simulink library "sm_ball_bearing_testrig_lib"  (R2019a)
settings: Solver=VariableStepAuto  StartTime=0.0  StopTime=10.0  RelTol=1e-3
undefined symbols (not defined in the file): bearing, bearing_ball_cage_b, bearing_ball_clr, bearing_ball_mark_clr, bearing_ball_mark_opc, bearing_ball_opc, bearing_ball_preload, bearing_ball_rad, bearing_ball_rho, bearing_cage_clr, bearing_cage_loop_xc, bearing_cage_opc, bearing_cage_rad_ctr, bearing_cage_rho, bearing_cage_web_thk, bearing_cage_web_xc, bearing_ir_all, bearing_ir_xc, bearing_or_all, bearing_or_xc, X, Y, Z
libraries: $bdroot x26, sm_lib x25, Contact_Forces_Lib x2, nesl_utility x1
Description:
  | Copyright 2018-2019 The MathWorks, Inc.
settings Model: Creator=smiller  LastModifiedBy=smiller
settings DataIOCC: ReturnWorkspaceOutputs=off
settings DebuggingCC: PregeneratedLibrarySubsystemCodeDiagnostic=none  ArithmeticOperatorsInVariantConditions=warning
settings SFSimCC: SimUseLocalCustomCode=off
settings RTWCC: RTWUseLocalCustomCode=off

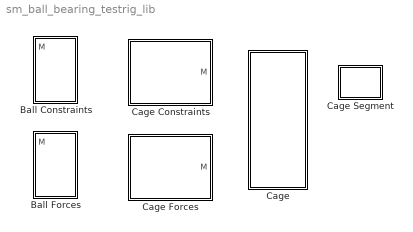
== system sm_ball_bearing_testrig_lib ==
  Ball Constraints : Subsystem  mask{ball_rad=0.005, ball_rho=7000, ball_cage_b=0, ball_clr=[0.6 0.6 0.6], ball_opc=1, mark_clr=[0.8 0.8 0.8], mark_opc=1, bearing_or=0.1, bearing_ir=0.05}
      mask prompts: ball_rad "Radius (m)"; ball_rho "Density (kg/m^3)"; ball_cage_b "Ball-Cage Viscous Friction (N*m/(deg/s))"; ball_clr "Color [R G B]"; ball_opc "Opacity (0-1)"; mark_clr "Color [R G B]"; mark_opc "Opacity (0-1)"; bearing_or "Bearing Outer Radius (m)"; bearing_ir "Bearing Inner Radius (m)"
      mask DialogControl cont_ball Prompt: Ball
      mask DialogControl cont_marking Prompt: Marking
      mask DialogControl cont_race Prompt: Race
      mask Display: image('sm_ball_bearing_testrig_ball_constraints_IMAGE.png');
  Ball Forces : Subsystem  mask{ball_rad=0.005, ball_rho=7000, ball_cage_b=0, ball_clr=[0.6 0.6 0.6], ball_opc=1, mark_clr=[0.8 0.8 0.8], mark_opc=1, bearing_or=0.1, bearing_ir=0.05, ball_k=1e5, ball_preload=5, ball_innerrace_overlap=0, ball_b=1e4, ball_muk=0.7, ball_mus=0.9, ball_vth=1e-3}
      mask prompts: ball_rad "Radius (m)"; ball_rho "Density (kg/m^3)"; ball_cage_b "Ball-Cage Viscous Friction (N*m/(deg/s))"; ball_clr "Color [RGB]"; ball_opc "Opacity (0-1)"; mark_clr "Color [RGB]"; mark_opc "Opacity (0-1)"; bearing_or "Bearing Outer Radius (m)"; bearing_ir "Bearing Inner Radius (m)"; ball_k "Stiffness (N/m)"; ball_preload "Preload Force Per Ball (N)"; ball_innerrace_overlap "Clearance (m)"; ball_b "Damping (N/(m/s))"; ball_muk "Coefficient of Kinetic Friction"; ball_mus "Coefficient of Static Friction"; ball_vth "Velocity Threshold (m/s)"
      mask init:
      | % Convert preload force to interference 
      | % for use in inner race contact force
      | % Positive interference = initial penetration
      | ball_innerrace_overlap = ball_preload/ball_k*2;
      mask DialogControl cont_ball Prompt: Ball
      mask DialogControl cont_marking Prompt: Marking
      mask DialogControl cont_race Prompt: Race
      mask DialogControl cont_forces Prompt: Forces
      mask Display: image('sm_ball_bearing_testrig_ball_forces_IMAGE.png');
  Cage : Subsystem
      mask Display: image('sm_ball_bearing_testrig_cage_IMAGE.png')
  Cage Constraints : Subsystem  Tag=PublishSubsystem  mask{ball_rad_all=bearing_ball_rad, ball_rho_all=bearing_ball_rho, ball_cage_b_all=bearing_ball_cage_b, ball_clr_all=bearing_ball_clr, ball_opc_all=bearing_ball_opc, ball_mark_clr_all=bearing_ball_mark_clr, ball_mark_opc_all=bearing_ball_mark_opc, bearing_or_all=max(bearing_or_xc(:,1))*2, bearing_ir_all=min(bearing_ir_xc(:,1))*2}
      mask prompts: ball_rad_all "Radius (m)"; ball_rho_all "Density (kg/m^3)"; ball_cage_b_all "Ball-Cage Viscous Friction (N*m/(deg/s))"; ball_clr_all "Color [R G B]"; ball_opc_all "Opacity (0-1)"; ball_mark_clr_all "Color [R G B]"; ball_mark_opc_all "Opacity (0-1)"; bearing_or_all "Bearing Outer Radius (m)"; bearing_ir_all "Bearing Inner Radius (m)"
      mask DialogControl cont_ball Prompt: Ball
      mask DialogControl cont_marking Prompt: Marking
      mask DialogControl cont_race_all Prompt: Race
      mask Display: image('sm_ball_bearing_testrig_cage_constraints_IMAGE.png');
  Cage Forces : Subsystem  Tag=PublishSubsystem  mask{ball_rad_all=bearing_ball_rad, ball_rho_all=bearing_ball_rho, ball_cage_b_all=bearing_ball_cage_b, ball_clr_all=bearing_ball_clr, ball_opc_all=bearing_ball_opc, ball_mark_clr_all=bearing_ball_mark_clr, ball_mark_opc_all=bearing_ball_mark_opc, bearing_or_all=max(bearing_or_xc(:,1))*2, bearing_ir_all=min(bearing_ir_xc(:,1))*2, ball_k_all=1e5, ball_preload_all=bearing_ball_preload, ball_b_all=1e4, ball_muk_all=0.7, ball_mus_all=0.9, ball_vth_all=1e-3}
      mask prompts: ball_rad_all "Radius (m)"; ball_rho_all "Density (kg/m^3)"; ball_cage_b_all "Ball-Cage Viscous Friction (N*m/(deg/s))"; ball_clr_all "Color [R G B]"; ball_opc_all "Opacity (0-1)"; ball_mark_clr_all "Color [R G B]"; ball_mark_opc_all "Opacity (0-1)"; bearing_or_all "Bearing Outer Radius (m)"; bearing_ir_all "Bearing Inner Radius (m)"; ball_k_all "Stiffness (N/m)"; ball_preload_all "Preload Force Per Ball (N)"; ball_b_all "Damping (N/(m/s))"; ball_muk_all "Coefficient of Kinetic Friction"; ball_mus_all "Coefficient of Static Friction"; ball_vth_all "Velocity Threshold (m/s)"
      mask DialogControl cont_ball Prompt: Ball
      mask DialogControl cont_marking Prompt: Marking
      mask DialogControl cont_race_all Prompt: Race
      mask DialogControl cont_forces Prompt: Forces
      mask Display: image('sm_ball_bearing_testrig_cage_forces_IMAGE.png');
  Cage Segment : Subsystem  mask{cage_loop_xc=bearing_cage_loop_xc, cage_web_xc=bearing_cage_web_xc, cage_web_thk=bearing_cage_web_thk, cage_rad_ctr=bearing_cage_rad_ctr, cage_rho=bearing_cage_rho, cage_clr=bearing_cage_clr, cage_opc=bearing_cage_opc}
      mask prompts: cage_loop_xc "Cross Section for Loop [x y] (m)"; cage_web_xc "Cross Section for Web [x y] (m)"; cage_web_thk "Thickness of Web (m)"; cage_rad_ctr "Radius of Web Centerline (m)"; cage_rho "Density (kg/m^3)"; cage_clr "Color [RGB]"; cage_opc "Opacity"
      mask DialogControl cont_cage Prompt: Cage
      mask Display: image('sm_ball_bearing_testrig_cage_segment_IMAGE.png')

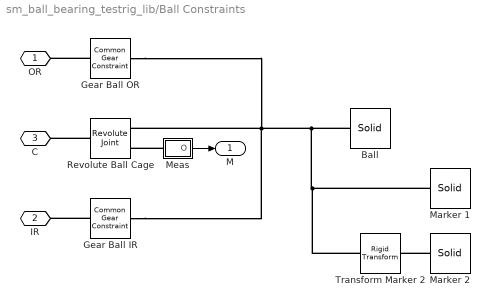
== system sm_ball_bearing_testrig_lib/Ball Constraints ==
  Ball : sm_lib/Body Elements/Solid  InertiaType=CalculateFromGeometry  Mass=1  MassUnits=kg  CenterOfMass=[0 0 0]  CenterOfMassUnits=m  MomentsOfInertia=[1 1 1]  MomentsOfInertiaUnits=kg*m^2  ProductsOfInertia=[1 1 1]  ProductsOfInertiaUnits=kg*m^2  BasedOnType=Density  Density=ball_rho  DensityUnits=kg/m^3  DoExposeReferenceFrame=on  SerializedFrames=<Frames/>  GraphicType=FromGeometry  MarkerShape=Sphere  MarkerSize=10  GraphicVisPropType=SimpleVisualProperties  GraphicDiffuseColor=ball_clr  GraphicSpecularColor=[0.5 0.5 0.5 1.0]  GraphicAmbientColor=[0.15 0.15 0.15 1.0]  GraphicEmissiveColor=[0.0 0.0 0.0 1.0]  GraphicShininess=75  GraphicOpacity=ball_opc  GeometryShape=Sphere  RectangleSize=[1 1]  RectangleSizeUnits=m  BrickDimensions=[1 1 1]  BrickDimensionUnits=m  CylinderRadius=1  CylinderRadiusUnits=m  CylinderLength=1  CylinderLengthUnits=m  SphereRadius=ball_rad  SphereRadiusUnits=m  EllipsoidRadii=[1 1 1]  EllipsoidRadiiUnits=m  ExtrusionCrossSection=[1 1; -1 1; -1 -1; 1 -1]  ExtrusionCrossSectionUnits=m  ExtrusionLength=1  ExtrusionLengthUnits=m  PolygonNumSides=3  PolygonOuterRadius=1  PolygonOuterRadiusUnits=m  ExtGeomFileType=STEP  ExtGeomFileUnits=m  RevolutionCrossSection=[1 1; 1 -1; 2 -1; 2 1]  RevolutionCrossSectionUnits=m  RevolutionExtent=Full  RevolutionAngle=180  RevolutionAngleUnits=deg
  Gear Ball IR : sm_lib/Gears and Couplings/Gears/Common Gear Constraint  GearType=External  SpecificationType=PitchCircleRadii  CenterDistance=20.0  CenterDistanceUnits=cm  GearRatio=1.0  BaseGearRadius=(bearing_or+bearing_ir)/4-ball_rad  BaseGearRadiusUnits=m  FollGearRadius=ball_rad  FollGearRadiusUnits=m  AssemblyGearRotation=Free
      settings: SourceProductName=Simscape Multibody  SourceProductBaseCode=MS
  Gear Ball OR : sm_lib/Gears and Couplings/Gears/Common Gear Constraint  GearType=Internal  SpecificationType=PitchCircleRadii  CenterDistance=20.0  CenterDistanceUnits=cm  GearRatio=1.0  BaseGearRadius=(bearing_or+bearing_ir)/4+ball_rad  BaseGearRadiusUnits=m  FollGearRadius=ball_rad  FollGearRadiusUnits=m  AssemblyGearRotation=Free
      settings: SourceProductName=Simscape Multibody  SourceProductBaseCode=MS
  Marker 1 : sm_lib/Body Elements/Solid  InertiaType=CalculateFromGeometry  Mass=1  MassUnits=kg  CenterOfMass=[0 0 0]  CenterOfMassUnits=m  MomentsOfInertia=[1 1 1]  MomentsOfInertiaUnits=kg*m^2  ProductsOfInertia=[1 1 1]  ProductsOfInertiaUnits=kg*m^2  BasedOnType=Density  Density=0  DensityUnits=kg/m^3  DoExposeReferenceFrame=on  SerializedFrames=<Frames/>  GraphicType=FromGeometry  MarkerShape=Sphere  MarkerSize=10  GraphicVisPropType=SimpleVisualProperties  GraphicDiffuseColor=mark_clr  GraphicSpecularColor=[0.5 0.5 0.5 1.0]  GraphicAmbientColor=[0.15 0.15 0.15 1.0]  GraphicEmissiveColor=[0.0 0.0 0.0 1.0]  GraphicShininess=75  GraphicOpacity=mark_opc  GeometryShape=GeneralSolidOfRevolution  RectangleSize=[1 1]  RectangleSizeUnits=m  BrickDimensions=[1 1 1]  BrickDimensionUnits=m  CylinderRadius=1  CylinderRadiusUnits=m  CylinderLength=1  CylinderLengthUnits=m  SphereRadius=1  SphereRadiusUnits=m  EllipsoidRadii=[1 1 1]  EllipsoidRadiiUnits=m  ExtrusionCrossSection=[1 1; -1 1; -1 -1; 1 -1]  ExtrusionCrossSectionUnits=m  ExtrusionLength=1  ExtrusionLengthUnits=m  PolygonNumSides=3  PolygonOuterRadius=1  PolygonOuterRadiusUnits=m  ExtGeomFileType=STEP  ExtGeomFileUnits=m  RevolutionCrossSection=[0.5 1; 0.5 -1; 0.7 -1; 0.7 1].*[ball_rad ball_rad*0.8]  RevolutionCrossSectionUnits=m  RevolutionExtent=Custom  RevolutionAngle=60  RevolutionAngleUnits=deg
  Marker 2 : sm_lib/Body Elements/Solid  InertiaType=CalculateFromGeometry  Mass=1  MassUnits=kg  CenterOfMass=[0 0 0]  CenterOfMassUnits=m  MomentsOfInertia=[1 1 1]  MomentsOfInertiaUnits=kg*m^2  ProductsOfInertia=[1 1 1]  ProductsOfInertiaUnits=kg*m^2  BasedOnType=Density  Density=0  DensityUnits=kg/m^3  DoExposeReferenceFrame=on  SerializedFrames=<Frames/>  GraphicType=FromGeometry  MarkerShape=Sphere  MarkerSize=10  GraphicVisPropType=SimpleVisualProperties  GraphicDiffuseColor=mark_clr  GraphicSpecularColor=[0.5 0.5 0.5 1.0]  GraphicAmbientColor=[0.15 0.15 0.15 1.0]  GraphicEmissiveColor=[0.0 0.0 0.0 1.0]  GraphicShininess=75  GraphicOpacity=mark_opc  GeometryShape=GeneralSolidOfRevolution  RectangleSize=[1 1]  RectangleSizeUnits=m  BrickDimensions=[1 1 1]  BrickDimensionUnits=m  CylinderRadius=1  CylinderRadiusUnits=m  CylinderLength=1  CylinderLengthUnits=m  SphereRadius=1  SphereRadiusUnits=m  EllipsoidRadii=[1 1 1]  EllipsoidRadiiUnits=m  ExtrusionCrossSection=[1 1; -1 1; -1 -1; 1 -1]  ExtrusionCrossSectionUnits=m  ExtrusionLength=1  ExtrusionLengthUnits=m  PolygonNumSides=3  PolygonOuterRadius=1  PolygonOuterRadiusUnits=m  ExtGeomFileType=STEP  ExtGeomFileUnits=m  RevolutionCrossSection=[0.5 1; 0.5 -1; 0.7 -1; 0.7 1].*[ball_rad ball_rad*0.8]  RevolutionCrossSectionUnits=m  RevolutionExtent=Custom  RevolutionAngle=60  RevolutionAngleUnits=deg
  Meas : Subsystem
  Revolute Ball Cage : sm_lib/Joints/Revolute Joint  SenseConstraintForce=off  SenseConstraintForceX=off  SenseConstraintForceY=off  SenseConstraintForceZ=off  SenseConstraintTorque=off  SenseConstraintTorqueX=off  SenseConstraintTorqueY=off  SenseConstraintTorqueZ=off  SenseTotalForce=off  SenseTotalForceX=off  SenseTotalForceY=off  SenseTotalForceZ=off  SenseTotalTorque=off  SenseTotalTorqueX=off  SenseTotalTorqueY=off  SenseTotalTorqueZ=off  CompositeWrenchDir=FollowerOnBase  CompositeWrenchFrame=BaseFrame  EquilibriumPosition=0  EquilibriumPositionUnits=deg  SpringStiffness=0  SpringStiffnessUnits=N*m/deg  DampingCoefficient=ball_cage_b  DampingCoefficientUnits=N*m/(deg/s)  TorqueActuationMode=NoTorque  MotionActuationMode=ComputedMotion  SensePosition=off  SenseVelocity=on  SenseAcceleration=off  SenseTorqueForce=off  SenseLowerLimitTorqueForce=off  SenseUpperLimitTorqueForce=off  LowerLimitSpecify=off  LowerLimitBound=-90  LowerLimitBoundUnits=deg  LowerLimitStiffness=1e4  LowerLimitStiffnessUnits=N*m/deg  LowerLimitDamping=10  LowerLimitDampingUnits=N*m/(deg/s)  LowerLimitTransitionRegionWidth=0.1  LowerLimitTransitionRegionWidthUnits=deg  UpperLimitSpecify=off  UpperLimitBound=90  UpperLimitBoundUnits=deg  UpperLimitStiffness=1e4  UpperLimitStiffnessUnits=N*m/deg  UpperLimitDamping=10  UpperLimitDampingUnits=N*m/(deg/s)  UpperLimitTransitionRegionWidth=0.1  UpperLimitTransitionRegionWidthUnits=deg  PositionTargetSpecify=off  PositionTargetPriority=High  PositionTargetValue=0  PositionTargetValueUnits=deg  VelocityTargetSpecify=off  VelocityTargetPriority=High  VelocityTargetValue=0  VelocityTargetValueUnits=deg/s
  Transform Marker 2 : sm_lib/Frames and Transforms/Rigid Transform  TranslationMethod=None  TranslationStandardOffset=0  TranslationLengthUnit=m  TranslationStandardAxis=+Z  TranslationCartesianOffset=[0 0 0]  TranslationROffset=0  TranslationROffsetUnits=m  TranslationZOffset=0  TranslationZOffsetUnits=m  TranslationThetaOffset=0  TranslationThetaOffsetUnits=deg  RotationMethod=StandardAxis  RotationAngleUnits=deg  RotationStandardAxis=+Z  RotationAngle=180  RotationArbitraryAxis=[0 0 1]  FollAlignAxisA=+X  BaseAlignAxisA=+Y  FollAlignAxisB=+Y  BaseAlignAxisB=+Z  RotationSequenceAxes=FollowerAxes  RotationSequence=XYX  RotationSequenceAngles=[0 0 0]  RotationSequenceAnglesUnits=deg  RotationMatrix=[1 0 0; 0 1 0; 0 0 1]
  OR : PMIOPort  Side=Right
  IR : PMIOPort  Port=2  Side=Right
  C : PMIOPort  Port=3  Side=Right
  M : Outport
  wires:
  Meas/1(O) -> M/1
  connections:
  Gear Ball OR/LConn1 -- OR/RConn1
  Gear Ball IR/LConn1 -- IR/RConn1
  Marker 1/RConn1 -- Ball/RConn1 -- Revolute Ball Cage/RConn1 -- Gear Ball OR/RConn1 -- Gear Ball IR/RConn1 -- Transform Marker 2/LConn1
  Revolute Ball Cage/LConn1 -- C/RConn1
  Marker 2/RConn1 -- Transform Marker 2/RConn1
  Meas/LConn1 -- Revolute Ball Cage/RConn2

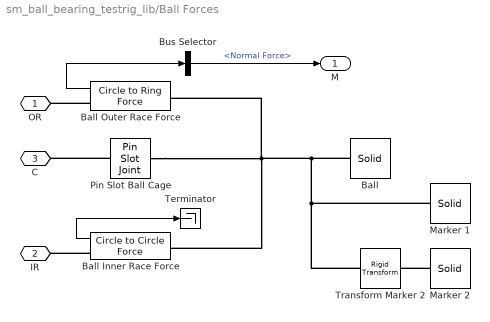
== system sm_ball_bearing_testrig_lib/Ball Forces ==
  Ball : sm_lib/Body Elements/Solid  InertiaType=CalculateFromGeometry  Mass=1  MassUnits=kg  CenterOfMass=[0 0 0]  CenterOfMassUnits=m  MomentsOfInertia=[1 1 1]  MomentsOfInertiaUnits=kg*m^2  ProductsOfInertia=[1 1 1]  ProductsOfInertiaUnits=kg*m^2  BasedOnType=Density  Density=ball_rho  DensityUnits=kg/m^3  DoExposeReferenceFrame=on  SerializedFrames=<Frames/>  GraphicType=FromGeometry  MarkerShape=Sphere  MarkerSize=10  GraphicVisPropType=SimpleVisualProperties  GraphicDiffuseColor=ball_clr  GraphicSpecularColor=[0.5 0.5 0.5 1.0]  GraphicAmbientColor=[0.15 0.15 0.15 1.0]  GraphicEmissiveColor=[0.0 0.0 0.0 1.0]  GraphicShininess=75  GraphicOpacity=ball_opc  GeometryShape=Sphere  RectangleSize=[1 1]  RectangleSizeUnits=m  BrickDimensions=[1 1 1]  BrickDimensionUnits=m  CylinderRadius=1  CylinderRadiusUnits=m  CylinderLength=1  CylinderLengthUnits=m  SphereRadius=ball_rad  SphereRadiusUnits=m  EllipsoidRadii=[1 1 1]  EllipsoidRadiiUnits=m  ExtrusionCrossSection=[1 1; -1 1; -1 -1; 1 -1]  ExtrusionCrossSectionUnits=m  ExtrusionLength=1  ExtrusionLengthUnits=m  PolygonNumSides=3  PolygonOuterRadius=1  PolygonOuterRadiusUnits=m  ExtGeomFileType=STEP  ExtGeomFileUnits=m  RevolutionCrossSection=[1 1; 1 -1; 2 -1; 2 1]  RevolutionCrossSectionUnits=m  RevolutionExtent=Full  RevolutionAngle=180  RevolutionAngleUnits=deg
  Ball Inner Race Force : Contact_Forces_Lib/2D/Circle to Circle Force  cirB_rad=(bearing_or+bearing_ir)/4-ball_rad+ball_innerrace_overlap  cirF_rad=ball_rad  active_angle=[-180 180]  force_law=Linear  k_contact=ball_k  b_contact=ball_b  pen_full_damp_F=1e-4  pen_exponent=1  custom_param_1=1  custom_param_2=1  friction_law=Stick-Slip Continuous  mu_kinetic=ball_muk  mu_static=ball_mus  v_thr=ball_vth  vis_on=off  vis_opc_en=0  vis_len_cirBz=0.1  vis_len_cirBx=0.005  vis_len_cirFz=0.1  vis_len_cirFx=0.005  vis_clr=[0.9 0.2 0.2]  vis_opc=0.7
      settings: SourceProductName=Simscape Multibody Contact Forces Library
  Ball Outer Race Force : Contact_Forces_Lib/2D/Circle to Ring Force  radius_circle=ball_rad  radius_ring=(bearing_or+bearing_ir)/4+ball_rad  d_ring=0  active_angle=[-180 180]  force_law=Linear  k_contact=ball_k  b_contact=ball_b  pen_full_damp_F=1e-4  pen_exponent=1  custom_param_1=1  custom_param_2=1  friction_law=Stick-Slip Continuous  mu_kinetic=ball_muk  mu_static=ball_mus  v_thr=ball_vth  vis_on=off  vis_opc_en=0  vis_len_rinBz=0.05*1.05  vis_len_rinBx=0.08*0.05  vis_len_cirFz=0.05*1.05  vis_len_cirFx=0.05*0.05  vis_clr=[0.9 0.2 0.2]  vis_opc=0.7
      settings: SourceProductName=Simscape Multibody Contact Forces Library
  Bus Selector : BusSelector  OutputSignals=Normal Force
  Marker 1 : sm_lib/Body Elements/Solid  InertiaType=CalculateFromGeometry  Mass=1  MassUnits=kg  CenterOfMass=[0 0 0]  CenterOfMassUnits=m  MomentsOfInertia=[1 1 1]  MomentsOfInertiaUnits=kg*m^2  ProductsOfInertia=[1 1 1]  ProductsOfInertiaUnits=kg*m^2  BasedOnType=Density  Density=0  DensityUnits=kg/m^3  DoExposeReferenceFrame=on  SerializedFrames=<Frames/>  GraphicType=FromGeometry  MarkerShape=Sphere  MarkerSize=10  GraphicVisPropType=SimpleVisualProperties  GraphicDiffuseColor=mark_clr  GraphicSpecularColor=[0.5 0.5 0.5 1.0]  GraphicAmbientColor=[0.15 0.15 0.15 1.0]  GraphicEmissiveColor=[0.0 0.0 0.0 1.0]  GraphicShininess=75  GraphicOpacity=mark_opc  GeometryShape=GeneralSolidOfRevolution  RectangleSize=[1 1]  RectangleSizeUnits=m  BrickDimensions=[1 1 1]  BrickDimensionUnits=m  CylinderRadius=1  CylinderRadiusUnits=m  CylinderLength=1  CylinderLengthUnits=m  SphereRadius=1  SphereRadiusUnits=m  EllipsoidRadii=[1 1 1]  EllipsoidRadiiUnits=m  ExtrusionCrossSection=[1 1; -1 1; -1 -1; 1 -1]  ExtrusionCrossSectionUnits=m  ExtrusionLength=1  ExtrusionLengthUnits=m  PolygonNumSides=3  PolygonOuterRadius=1  PolygonOuterRadiusUnits=m  ExtGeomFileType=STEP  ExtGeomFileUnits=m  RevolutionCrossSection=[0.5 1; 0.5 -1; 0.7 -1; 0.7 1].*[ball_rad ball_rad*0.8]  RevolutionCrossSectionUnits=m  RevolutionExtent=Custom  RevolutionAngle=60  RevolutionAngleUnits=deg
  Marker 2 : sm_lib/Body Elements/Solid  InertiaType=CalculateFromGeometry  Mass=1  MassUnits=kg  CenterOfMass=[0 0 0]  CenterOfMassUnits=m  MomentsOfInertia=[1 1 1]  MomentsOfInertiaUnits=kg*m^2  ProductsOfInertia=[1 1 1]  ProductsOfInertiaUnits=kg*m^2  BasedOnType=Density  Density=0  DensityUnits=kg/m^3  DoExposeReferenceFrame=on  SerializedFrames=<Frames/>  GraphicType=FromGeometry  MarkerShape=Sphere  MarkerSize=10  GraphicVisPropType=SimpleVisualProperties  GraphicDiffuseColor=mark_clr  GraphicSpecularColor=[0.5 0.5 0.5 1.0]  GraphicAmbientColor=[0.15 0.15 0.15 1.0]  GraphicEmissiveColor=[0.0 0.0 0.0 1.0]  GraphicShininess=75  GraphicOpacity=mark_opc  GeometryShape=GeneralSolidOfRevolution  RectangleSize=[1 1]  RectangleSizeUnits=m  BrickDimensions=[1 1 1]  BrickDimensionUnits=m  CylinderRadius=1  CylinderRadiusUnits=m  CylinderLength=1  CylinderLengthUnits=m  SphereRadius=1  SphereRadiusUnits=m  EllipsoidRadii=[1 1 1]  EllipsoidRadiiUnits=m  ExtrusionCrossSection=[1 1; -1 1; -1 -1; 1 -1]  ExtrusionCrossSectionUnits=m  ExtrusionLength=1  ExtrusionLengthUnits=m  PolygonNumSides=3  PolygonOuterRadius=1  PolygonOuterRadiusUnits=m  ExtGeomFileType=STEP  ExtGeomFileUnits=m  RevolutionCrossSection=[0.5 1; 0.5 -1; 0.7 -1; 0.7 1].*[ball_rad ball_rad*0.8]  RevolutionCrossSectionUnits=m  RevolutionExtent=Custom  RevolutionAngle=60  RevolutionAngleUnits=deg
  Pin Slot Ball Cage : sm_lib/Joints/Pin Slot Joint  SenseConstraintForce=off  SenseConstraintForceX=off  SenseConstraintForceY=off  SenseConstraintForceZ=off  SenseConstraintTorque=off  SenseConstraintTorqueX=off  SenseConstraintTorqueY=off  SenseConstraintTorqueZ=off  SenseTotalForce=off  SenseTotalForceX=off  SenseTotalForceY=off  SenseTotalForceZ=off  SenseTotalTorque=off  SenseTotalTorqueX=off  SenseTotalTorqueY=off  SenseTotalTorqueZ=off  CompositeWrenchDir=FollowerOnBase  CompositeWrenchFrame=BaseFrame  PxEquilibriumPosition=0  PxEquilibriumPositionUnits=m  PxSpringStiffness=0  PxSpringStiffnessUnits=N/m  PxDampingCoefficient=0  PxDampingCoefficientUnits=N/(m/s)  PxTorqueActuationMode=NoTorque  PxMotionActuationMode=ComputedMotion  PxSensePosition=off  PxSenseVelocity=off  PxSenseAcceleration=off  PxSenseTorqueForce=off  PxSenseLowerLimitTorqueForce=off  PxSenseUpperLimitTorqueForce=off  PxLowerLimitSpecify=off  PxLowerLimitBound=-1  PxLowerLimitBoundUnits=m  PxLowerLimitStiffness=1e6  PxLowerLimitStiffnessUnits=N/m  PxLowerLimitDamping=1e3  PxLowerLimitDampingUnits=N/(m/s)  PxLowerLimitTransitionRegionWidth=1e-4  PxLowerLimitTransitionRegionWidthUnits=m  PxUpperLimitSpecify=off  PxUpperLimitBound=1  PxUpperLimitBoundUnits=m  PxUpperLimitStiffness=1e6  PxUpperLimitStiffnessUnits=N/m  PxUpperLimitDamping=1e3  PxUpperLimitDampingUnits=N/(m/s)  PxUpperLimitTransitionRegionWidth=1e-4  PxUpperLimitTransitionRegionWidthUnits=m  PxPositionTargetSpecify=on  PxPositionTargetPriority=High  PxPositionTargetValue=ball_innerrace_overlap/2  PxPositionTargetValueUnits=m  PxVelocityTargetSpecify=off  PxVelocityTargetPriority=High  PxVelocityTargetValue=0  PxVelocityTargetValueUnits=m/s  RzEquilibriumPosition=0  RzEquilibriumPositionUnits=deg  RzSpringStiffness=0  RzSpringStiffnessUnits=N*m/deg  RzDampingCoefficient=ball_cage_b  RzDampingCoefficientUnits=N*m/(deg/s)  RzTorqueActuationMode=NoTorque  RzMotionActuationMode=ComputedMotion  RzSensePosition=off  RzSenseVelocity=off  RzSenseAcceleration=off  RzSenseTorqueForce=off  RzSenseLowerLimitTorqueForce=off  RzSenseUpperLimitTorqueForce=off  RzLowerLimitSpecify=off  RzLowerLimitBound=-90  RzLowerLimitBoundUnits=deg  RzLowerLimitStiffness=1e4  RzLowerLimitStiffnessUnits=N*m/deg  RzLowerLimitDamping=10  RzLowerLimitDampingUnits=N*m/(deg/s)  RzLowerLimitTransitionRegionWidth=0.1  RzLowerLimitTransitionRegionWidthUnits=deg  RzUpperLimitSpecify=off  RzUpperLimitBound=90  RzUpperLimitBoundUnits=deg  RzUpperLimitStiffness=1e4  RzUpperLimitStiffnessUnits=N*m/deg  RzUpperLimitDamping=10  RzUpperLimitDampingUnits=N*m/(deg/s)  RzUpperLimitTransitionRegionWidth=0.1  RzUpperLimitTransitionRegionWidthUnits=deg  RzPositionTargetSpecify=off  RzPositionTargetPriority=High  RzPositionTargetValue=0  RzPositionTargetValueUnits=deg  RzVelocityTargetSpecify=off  RzVelocityTargetPriority=High  RzVelocityTargetValue=0  RzVelocityTargetValueUnits=deg/s
      settings: SourceProductName=Simscape Multibody  SourceProductBaseCode=MS
  Terminator : Terminator
  Transform Marker 2 : sm_lib/Frames and Transforms/Rigid Transform  TranslationMethod=None  TranslationStandardOffset=0  TranslationLengthUnit=m  TranslationStandardAxis=+Z  TranslationCartesianOffset=[0 0 0]  TranslationROffset=0  TranslationROffsetUnits=m  TranslationZOffset=0  TranslationZOffsetUnits=m  TranslationThetaOffset=0  TranslationThetaOffsetUnits=deg  RotationMethod=StandardAxis  RotationAngleUnits=deg  RotationStandardAxis=+Z  RotationAngle=180  RotationArbitraryAxis=[0 0 1]  FollAlignAxisA=+X  BaseAlignAxisA=+Y  FollAlignAxisB=+Y  BaseAlignAxisB=+Z  RotationSequenceAxes=FollowerAxes  RotationSequence=XYX  RotationSequenceAngles=[0 0 0]  RotationSequenceAnglesUnits=deg  RotationMatrix=[1 0 0; 0 1 0; 0 0 1]
  OR : PMIOPort  Side=Right
  IR : PMIOPort  Port=2  Side=Right
  C : PMIOPort  Port=3  Side=Right
  M : Outport
  wires:
  Bus Selector/1 -> M/1  "<Normal Force>"
  Ball Outer Race Force/1 -> Bus Selector/1
  Ball Inner Race Force/1 -> Terminator/1
  connections:
  Marker 2/RConn1 -- Transform Marker 2/RConn1
  Pin Slot Ball Cage/LConn1 -- C/RConn1
  Transform Marker 2/LConn1 -- Marker 1/RConn1 -- Pin Slot Ball Cage/RConn1 -- Ball Inner Race Force/LConn1 -- Ball Outer Race Force/LConn1 -- Ball/RConn1
  Ball Inner Race Force/RConn1 -- IR/RConn1
  Ball Outer Race Force/RConn1 -- OR/RConn1

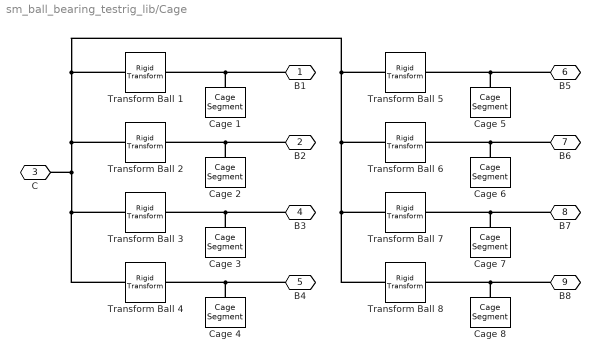
== system sm_ball_bearing_testrig_lib/Cage ==
  Cage {1..8} (8 alike) : $bdroot/Cage Segment  cage_loop_xc=bearing_cage_loop_xc  cage_web_xc=bearing_cage_web_xc  cage_web_thk=bearing_cage_web_thk  cage_rad_ctr=bearing_cage_rad_ctr  cage_rho=bearing_cage_rho  cage_clr=bearing_cage_clr  cage_opc=bearing_cage_opc
  Transform Ball 1 : sm_lib/Frames and Transforms/Rigid Transform  TranslationMethod=Cylindrical  TranslationStandardOffset=0  TranslationLengthUnit=m  TranslationStandardAxis=+Z  TranslationCartesianOffset=[0 0 0]  TranslationROffset=(bearing.D+bearing.d)/4  TranslationROffsetUnits=m  TranslationZOffset=0  TranslationZOffsetUnits=m  TranslationThetaOffset=0  TranslationThetaOffsetUnits=deg  RotationMethod=None  RotationAngleUnits=deg  RotationStandardAxis=+Z  RotationAngle=0.0  RotationArbitraryAxis=[0 0 1]  FollAlignAxisA=+X  BaseAlignAxisA=+Y  FollAlignAxisB=+Y  BaseAlignAxisB=+Z  RotationSequenceAxes=FollowerAxes  RotationSequence=XYX  RotationSequenceAngles=[0 0 0]  RotationSequenceAnglesUnits=deg  RotationMatrix=[1 0 0; 0 1 0; 0 0 1]
  Transform Ball 2 : sm_lib/Frames and Transforms/Rigid Transform  TranslationMethod=Cylindrical  TranslationStandardOffset=0  TranslationLengthUnit=m  TranslationStandardAxis=+Z  TranslationCartesianOffset=[0 0 0]  TranslationROffset=(bearing.D+bearing.d)/4  TranslationROffsetUnits=m  TranslationZOffset=0  TranslationZOffsetUnits=m  TranslationThetaOffset=360/8  TranslationThetaOffsetUnits=deg  RotationMethod=StandardAxis  RotationAngleUnits=deg  RotationStandardAxis=+Z  RotationAngle=360/8  RotationArbitraryAxis=[0 0 1]  FollAlignAxisA=+X  BaseAlignAxisA=+Y  FollAlignAxisB=+Y  BaseAlignAxisB=+Z  RotationSequenceAxes=FollowerAxes  RotationSequence=XYX  RotationSequenceAngles=[0 0 0]  RotationSequenceAnglesUnits=deg  RotationMatrix=[1 0 0; 0 1 0; 0 0 1]
  Transform Ball 3 : sm_lib/Frames and Transforms/Rigid Transform  TranslationMethod=Cylindrical  TranslationStandardOffset=0  TranslationLengthUnit=m  TranslationStandardAxis=+Z  TranslationCartesianOffset=[0 0 0]  TranslationROffset=(bearing.D+bearing.d)/4  TranslationROffsetUnits=m  TranslationZOffset=0  TranslationZOffsetUnits=m  TranslationThetaOffset=360/8*2  TranslationThetaOffsetUnits=deg  RotationMethod=StandardAxis  RotationAngleUnits=deg  RotationStandardAxis=+Z  RotationAngle=360/8*2  RotationArbitraryAxis=[0 0 1]  FollAlignAxisA=+X  BaseAlignAxisA=+Y  FollAlignAxisB=+Y  BaseAlignAxisB=+Z  RotationSequenceAxes=FollowerAxes  RotationSequence=XYX  RotationSequenceAngles=[0 0 0]  RotationSequenceAnglesUnits=deg  RotationMatrix=[1 0 0; 0 1 0; 0 0 1]
  Transform Ball 4 : sm_lib/Frames and Transforms/Rigid Transform  TranslationMethod=Cylindrical  TranslationStandardOffset=0  TranslationLengthUnit=m  TranslationStandardAxis=+Z  TranslationCartesianOffset=[0 0 0]  TranslationROffset=(bearing.D+bearing.d)/4  TranslationROffsetUnits=m  TranslationZOffset=0  TranslationZOffsetUnits=m  TranslationThetaOffset=360/8*3  TranslationThetaOffsetUnits=deg  RotationMethod=StandardAxis  RotationAngleUnits=deg  RotationStandardAxis=+Z  RotationAngle=360/8*3  RotationArbitraryAxis=[0 0 1]  FollAlignAxisA=+X  BaseAlignAxisA=+Y  FollAlignAxisB=+Y  BaseAlignAxisB=+Z  RotationSequenceAxes=FollowerAxes  RotationSequence=XYX  RotationSequenceAngles=[0 0 0]  RotationSequenceAnglesUnits=deg  RotationMatrix=[1 0 0; 0 1 0; 0 0 1]
  Transform Ball 5 : sm_lib/Frames and Transforms/Rigid Transform  TranslationMethod=Cylindrical  TranslationStandardOffset=0  TranslationLengthUnit=m  TranslationStandardAxis=+Z  TranslationCartesianOffset=[0 0 0]  TranslationROffset=(bearing.D+bearing.d)/4  TranslationROffsetUnits=m  TranslationZOffset=0  TranslationZOffsetUnits=m  TranslationThetaOffset=360/8*4  TranslationThetaOffsetUnits=deg  RotationMethod=StandardAxis  RotationAngleUnits=deg  RotationStandardAxis=+Z  RotationAngle=360/8*4  RotationArbitraryAxis=[0 0 1]  FollAlignAxisA=+X  BaseAlignAxisA=+Y  FollAlignAxisB=+Y  BaseAlignAxisB=+Z  RotationSequenceAxes=FollowerAxes  RotationSequence=XYX  RotationSequenceAngles=[0 0 0]  RotationSequenceAnglesUnits=deg  RotationMatrix=[1 0 0; 0 1 0; 0 0 1]
  Transform Ball 6 : sm_lib/Frames and Transforms/Rigid Transform  TranslationMethod=Cylindrical  TranslationStandardOffset=0  TranslationLengthUnit=m  TranslationStandardAxis=+Z  TranslationCartesianOffset=[0 0 0]  TranslationROffset=(bearing.D+bearing.d)/4  TranslationROffsetUnits=m  TranslationZOffset=0  TranslationZOffsetUnits=m  TranslationThetaOffset=360/8*5  TranslationThetaOffsetUnits=deg  RotationMethod=StandardAxis  RotationAngleUnits=deg  RotationStandardAxis=+Z  RotationAngle=360/8*5  RotationArbitraryAxis=[0 0 1]  FollAlignAxisA=+X  BaseAlignAxisA=+Y  FollAlignAxisB=+Y  BaseAlignAxisB=+Z  RotationSequenceAxes=FollowerAxes  RotationSequence=XYX  RotationSequenceAngles=[0 0 0]  RotationSequenceAnglesUnits=deg  RotationMatrix=[1 0 0; 0 1 0; 0 0 1]
  Transform Ball 7 : sm_lib/Frames and Transforms/Rigid Transform  TranslationMethod=Cylindrical  TranslationStandardOffset=0  TranslationLengthUnit=m  TranslationStandardAxis=+Z  TranslationCartesianOffset=[0 0 0]  TranslationROffset=(bearing.D+bearing.d)/4  TranslationROffsetUnits=m  TranslationZOffset=0  TranslationZOffsetUnits=m  TranslationThetaOffset=360/8*6  TranslationThetaOffsetUnits=deg  RotationMethod=StandardAxis  RotationAngleUnits=deg  RotationStandardAxis=+Z  RotationAngle=360/8*6  RotationArbitraryAxis=[0 0 1]  FollAlignAxisA=+X  BaseAlignAxisA=+Y  FollAlignAxisB=+Y  BaseAlignAxisB=+Z  RotationSequenceAxes=FollowerAxes  RotationSequence=XYX  RotationSequenceAngles=[0 0 0]  RotationSequenceAnglesUnits=deg  RotationMatrix=[1 0 0; 0 1 0; 0 0 1]
  Transform Ball 8 : sm_lib/Frames and Transforms/Rigid Transform  TranslationMethod=Cylindrical  TranslationStandardOffset=0  TranslationLengthUnit=m  TranslationStandardAxis=+Z  TranslationCartesianOffset=[0 0 0]  TranslationROffset=(bearing.D+bearing.d)/4  TranslationROffsetUnits=m  TranslationZOffset=0  TranslationZOffsetUnits=m  TranslationThetaOffset=360/8*7  TranslationThetaOffsetUnits=deg  RotationMethod=StandardAxis  RotationAngleUnits=deg  RotationStandardAxis=+Z  RotationAngle=360/8*7  RotationArbitraryAxis=[0 0 1]  FollAlignAxisA=+X  BaseAlignAxisA=+Y  FollAlignAxisB=+Y  BaseAlignAxisB=+Z  RotationSequenceAxes=FollowerAxes  RotationSequence=XYX  RotationSequenceAngles=[0 0 0]  RotationSequenceAnglesUnits=deg  RotationMatrix=[1 0 0; 0 1 0; 0 0 1]
  B1 : PMIOPort  Side=Right
  B2 : PMIOPort  Port=2  Side=Right
  C : PMIOPort  Port=3  Side=Left
  B3 : PMIOPort  Port=4  Side=Right
  B4 : PMIOPort  Port=5  Side=Right
  B5 : PMIOPort  Port=6  Side=Right
  B6 : PMIOPort  Port=7  Side=Right
  B7 : PMIOPort  Port=8  Side=Right
  B8 : PMIOPort  Port=9  Side=Right
  connections:
  Transform Ball 8/RConn1 -- B8/RConn1 -- Cage 8/LConn1
  Transform Ball 7/RConn1 -- B7/RConn1 -- Cage 7/LConn1
  Transform Ball 6/RConn1 -- B6/RConn1 -- Cage 6/LConn1
  Transform Ball 5/RConn1 -- B5/RConn1 -- Cage 5/LConn1
  Transform Ball 4/RConn1 -- B4/RConn1 -- Cage 4/LConn1
  Transform Ball 3/RConn1 -- B3/RConn1 -- Cage 3/LConn1
  Transform Ball 2/RConn1 -- B2/RConn1 -- Cage 2/LConn1
  B1/RConn1 -- Cage 1/LConn1 -- Transform Ball 1/RConn1
  Transform Ball 2/LConn1 -- C/RConn1 -- Transform Ball 3/LConn1 -- Transform Ball 4/LConn1 -- Transform Ball 7/LConn1 -- Transform Ball 8/LConn1 -- Transform Ball 6/LConn1 -- Transform Ball 5/LConn1 -- Transform Ball 1/LConn1

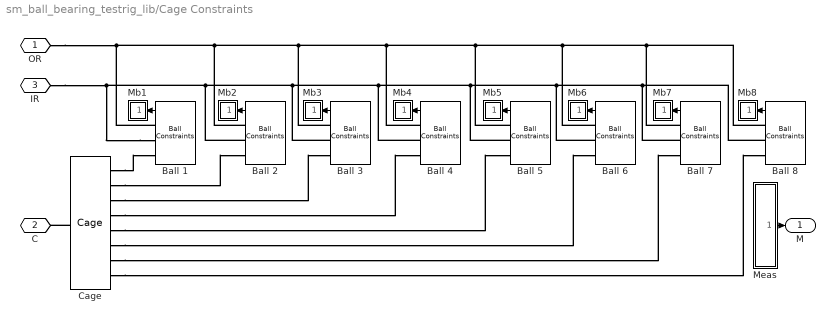
== system sm_ball_bearing_testrig_lib/Cage Constraints ==
  Ball 1 : $bdroot/Ball Constraints  Tag=PublishSubsystem  ball_rad=ball_rad_all  ball_rho=ball_rho_all  ball_cage_b=ball_cage_b_all  ball_clr=ball_clr_all  ball_opc=ball_opc_all  mark_clr=ball_mark_clr_all  mark_opc=ball_mark_opc_all  bearing_or=bearing_or_all  bearing_ir=bearing_ir_all
  Ball {2..8} (7 alike) : $bdroot/Ball Constraints  ball_rad=ball_rad_all  ball_rho=ball_rho_all  ball_cage_b=ball_cage_b_all  ball_clr=ball_clr_all  ball_opc=ball_opc_all  mark_clr=ball_mark_clr_all  mark_opc=ball_mark_opc_all  bearing_or=bearing_or_all  bearing_ir=bearing_ir_all
  Cage : $bdroot/Cage  SystemSampleTime=-1
  Mb1 : Subsystem
  Mb2 : Subsystem
  Mb3 : Subsystem
  Mb4 : Subsystem
  Mb5 : Subsystem
  Mb6 : Subsystem
  Mb7 : Subsystem
  Mb8 : Subsystem
  Meas : Subsystem
  OR : PMIOPort  Side=Left
  C : PMIOPort  Port=2  Side=Left
  IR : PMIOPort  Port=3  Side=Left
  M : Outport
  wires:
  Ball 8/1 -> Mb8/1(M)
  Ball 7/1 -> Mb7/1(M)
  Ball 6/1 -> Mb6/1(M)
  Ball 5/1 -> Mb5/1(M)
  Ball 4/1 -> Mb4/1(M)
  Ball 3/1 -> Mb3/1(M)
  Ball 2/1 -> Mb2/1(M)
  Ball 1/1 -> Mb1/1(M)
  Meas/1(M) -> M/1
  connections:
  Cage/RConn8 -- Ball 8/RConn3
  Cage/RConn7 -- Ball 7/RConn3
  Cage/RConn6 -- Ball 6/RConn3
  Cage/RConn5 -- Ball 5/RConn3
  Cage/RConn4 -- Ball 4/RConn3
  Cage/RConn3 -- Ball 3/RConn3
  Cage/RConn2 -- Ball 2/RConn3
  Cage/RConn1 -- Ball 1/RConn3
  Ball 1/RConn2 -- Ball 2/RConn2 -- Ball 3/RConn2 -- Ball 4/RConn2 -- Ball 5/RConn2 -- Ball 6/RConn2 -- Ball 7/RConn2 -- Ball 8/RConn2 -- IR/RConn1
  Cage/LConn1 -- C/RConn1
  Ball 5/RConn1 -- OR/RConn1 -- Ball 1/RConn1 -- Ball 2/RConn1 -- Ball 3/RConn1 -- Ball 4/RConn1 -- Ball 6/RConn1 -- Ball 7/RConn1 -- Ball 8/RConn1

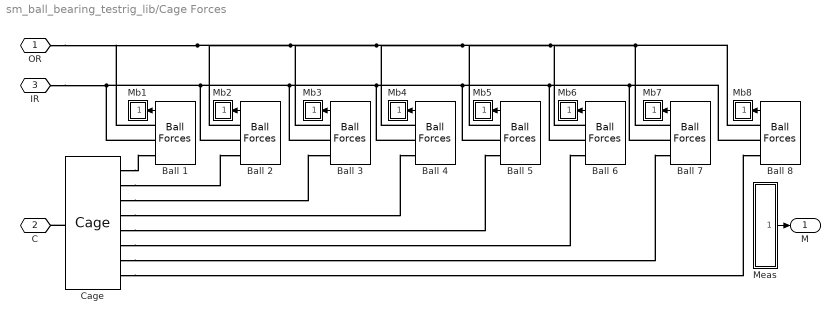
== system sm_ball_bearing_testrig_lib/Cage Forces ==
  Ball 1 : $bdroot/Ball Forces  Tag=PublishSubsystem  ball_rad=ball_rad_all  ball_rho=ball_rho_all  ball_cage_b=ball_cage_b_all  ball_clr=ball_clr_all  ball_opc=ball_opc_all  mark_clr=ball_mark_clr_all  mark_opc=ball_mark_opc_all  bearing_or=bearing_or_all  bearing_ir=bearing_ir_all  ball_k=ball_k_all  ball_preload=ball_preload_all  ball_innerrace_overlap=0  ball_b=ball_b_all  ball_muk=ball_muk_all  ball_mus=ball_mus_all  ball_vth=ball_vth_all
  Ball 2 : $bdroot/Ball Forces  ball_rad=ball_rad_all  ball_rho=ball_rho_all  ball_cage_b=ball_cage_b_all  ball_clr=ball_clr_all  ball_opc=ball_opc_all  mark_clr=ball_mark_clr_all  mark_opc=ball_mark_opc_all  bearing_or=bearing_or_all  bearing_ir=bearing_ir_all  ball_k=ball_k_all  ball_preload=ball_preload_all  ball_innerrace_overlap=0  ball_b=ball_b_all  ball_muk=ball_muk_all  ball_mus=0.9  ball_vth=ball_vth_all
  Ball {3..8} (6 alike) : $bdroot/Ball Forces  ball_rad=ball_rad_all  ball_rho=ball_rho_all  ball_cage_b=ball_cage_b_all  ball_clr=ball_clr_all  ball_opc=ball_opc_all  mark_clr=ball_mark_clr_all  mark_opc=ball_mark_opc_all  bearing_or=bearing_or_all  bearing_ir=bearing_ir_all  ball_k=ball_k_all  ball_preload=ball_preload_all  ball_innerrace_overlap=0  ball_b=ball_b_all  ball_muk=ball_muk_all  ball_mus=ball_mus_all  ball_vth=ball_vth_all
  Cage : $bdroot/Cage  SystemSampleTime=-1
  Mb1 : Subsystem
  Mb2 : Subsystem
  Mb3 : Subsystem
  Mb4 : Subsystem
  Mb5 : Subsystem
  Mb6 : Subsystem
  Mb7 : Subsystem
  Mb8 : Subsystem
  Meas : Subsystem
  OR : PMIOPort  Side=Left
  C : PMIOPort  Port=2  Side=Left
  IR : PMIOPort  Port=3  Side=Left
  M : Outport
  wires:
  Ball 8/1 -> Mb8/1(M)
  Ball 7/1 -> Mb7/1(M)
  Ball 6/1 -> Mb6/1(M)
  Ball 5/1 -> Mb5/1(M)
  Ball 4/1 -> Mb4/1(M)
  Ball 3/1 -> Mb3/1(M)
  Ball 2/1 -> Mb2/1(M)
  Ball 1/1 -> Mb1/1(M)
  Meas/1(M) -> M/1
  connections:
  Cage/RConn8 -- Ball 8/RConn3
  Cage/RConn7 -- Ball 7/RConn3
  Cage/RConn6 -- Ball 6/RConn3
  Cage/RConn5 -- Ball 5/RConn3
  Cage/RConn4 -- Ball 4/RConn3
  Cage/RConn3 -- Ball 3/RConn3
  Cage/RConn2 -- Ball 2/RConn3
  Cage/RConn1 -- Ball 1/RConn3
  Ball 8/RConn2 -- Ball 4/RConn2 -- Ball 3/RConn2 -- IR/RConn1 -- Ball 1/RConn2 -- Ball 2/RConn2 -- Ball 5/RConn2 -- Ball 6/RConn2 -- Ball 7/RConn2
  Cage/LConn1 -- C/RConn1
  Ball 8/RConn1 -- Ball 7/RConn1 -- Ball 5/RConn1 -- Ball 4/RConn1 -- Ball 2/RConn1 -- OR/RConn1 -- Ball 1/RConn1 -- Ball 3/RConn1 -- Ball 6/RConn1

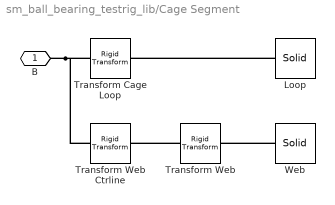
== system sm_ball_bearing_testrig_lib/Cage Segment ==
  Loop : sm_lib/Body Elements/Solid  InertiaType=CalculateFromGeometry  Mass=1  MassUnits=kg  CenterOfMass=[0 0 0]  CenterOfMassUnits=m  MomentsOfInertia=[1 1 1]  MomentsOfInertiaUnits=kg*m^2  ProductsOfInertia=[1 1 1]  ProductsOfInertiaUnits=kg*m^2  BasedOnType=Density  Density=cage_rho  DensityUnits=kg/m^3  DoExposeReferenceFrame=on  SerializedFrames=<Frames/>  GraphicType=FromGeometry  MarkerShape=Sphere  MarkerSize=10  GraphicVisPropType=SimpleVisualProperties  GraphicDiffuseColor=cage_clr  GraphicSpecularColor=[0.5 0.5 0.5 1.0]  GraphicAmbientColor=[0.15 0.15 0.15 1.0]  GraphicEmissiveColor=[0.0 0.0 0.0 1.0]  GraphicShininess=75  GraphicOpacity=cage_opc  GeometryShape=GeneralSolidOfRevolution  RectangleSize=[1 1]  RectangleSizeUnits=m  BrickDimensions=[1 1 1]  BrickDimensionUnits=m  CylinderRadius=1  CylinderRadiusUnits=m  CylinderLength=1  CylinderLengthUnits=m  SphereRadius=1  SphereRadiusUnits=m  EllipsoidRadii=[1 1 1]  EllipsoidRadiiUnits=m  ExtrusionCrossSection=[1 1; -1 1; -1 -1; 1 -1]  ExtrusionCrossSectionUnits=m  ExtrusionLength=1  ExtrusionLengthUnits=m  PolygonNumSides=3  PolygonOuterRadius=1  PolygonOuterRadiusUnits=m  ExtGeomFileType=STEP  ExtGeomFileUnits=m  RevolutionCrossSection=cage_loop_xc  RevolutionCrossSectionUnits=m  RevolutionExtent=Full  RevolutionAngle=180  RevolutionAngleUnits=deg
  Transform Cage Loop : sm_lib/Frames and Transforms/Rigid Transform  TranslationMethod=None  TranslationStandardOffset=0  TranslationLengthUnit=m  TranslationStandardAxis=+Z  TranslationCartesianOffset=[0 0 0]  TranslationROffset=0  TranslationROffsetUnits=m  TranslationZOffset=0  TranslationZOffsetUnits=m  TranslationThetaOffset=0  TranslationThetaOffsetUnits=deg  RotationMethod=StandardAxis  RotationAngleUnits=deg  RotationStandardAxis=+Y  RotationAngle=-90  RotationArbitraryAxis=[0 0 1]  FollAlignAxisA=+X  BaseAlignAxisA=+Y  FollAlignAxisB=+Y  BaseAlignAxisB=+Z  RotationSequenceAxes=FollowerAxes  RotationSequence=XYX  RotationSequenceAngles=[0 0 0]  RotationSequenceAnglesUnits=deg  RotationMatrix=[1 0 0; 0 1 0; 0 0 1]
  Transform Web : sm_lib/Frames and Transforms/Rigid Transform  TranslationMethod=Cartesian  TranslationStandardOffset=0  TranslationLengthUnit=m  TranslationStandardAxis=+Z  TranslationCartesianOffset=[-(1-cosd(360/8/2)) sind(360/8/2) 0]*cage_rad_ctr  TranslationROffset=0  TranslationROffsetUnits=m  TranslationZOffset=0  TranslationZOffsetUnits=m  TranslationThetaOffset=0  TranslationThetaOffsetUnits=deg  RotationMethod=StandardAxis  RotationAngleUnits=deg  RotationStandardAxis=+Z  RotationAngle=360/8/2  RotationArbitraryAxis=[0 0 1]  FollAlignAxisA=+X  BaseAlignAxisA=+Y  FollAlignAxisB=+Y  BaseAlignAxisB=+Z  RotationSequenceAxes=FollowerAxes  RotationSequence=XYX  RotationSequenceAngles=[0 0 0]  RotationSequenceAnglesUnits=deg  RotationMatrix=[1 0 0; 0 1 0; 0 0 1]
  Transform Web Ctrline : sm_lib/Frames and Transforms/Rigid Transform  TranslationMethod=StandardAxis  TranslationStandardOffset=cage_rad_ctr-(bearing_or_all+bearing_ir_all)/4  TranslationLengthUnit=m  TranslationStandardAxis=+X  TranslationCartesianOffset=[0 0 0]  TranslationROffset=0  TranslationROffsetUnits=m  TranslationZOffset=0  TranslationZOffsetUnits=m  TranslationThetaOffset=0  TranslationThetaOffsetUnits=deg  RotationMethod=None  RotationAngleUnits=deg  RotationStandardAxis=+Z  RotationAngle=0  RotationArbitraryAxis=[0 0 1]  FollAlignAxisA=+X  BaseAlignAxisA=+Y  FollAlignAxisB=+Y  BaseAlignAxisB=+Z  RotationSequenceAxes=FollowerAxes  RotationSequence=XYX  RotationSequenceAngles=[0 0 0]  RotationSequenceAnglesUnits=deg  RotationMatrix=[1 0 0; 0 1 0; 0 0 1]
  Web : sm_lib/Body Elements/Solid  InertiaType=CalculateFromGeometry  Mass=1  MassUnits=kg  CenterOfMass=[0 0 0]  CenterOfMassUnits=m  MomentsOfInertia=[1 1 1]  MomentsOfInertiaUnits=kg*m^2  ProductsOfInertia=[1 1 1]  ProductsOfInertiaUnits=kg*m^2  BasedOnType=Density  Density=cage_rho  DensityUnits=kg/m^3  DoExposeReferenceFrame=on  SerializedFrames=<Frames/>  GraphicType=FromGeometry  MarkerShape=Sphere  MarkerSize=10  GraphicVisPropType=SimpleVisualProperties  GraphicDiffuseColor=cage_clr  GraphicSpecularColor=[0.5 0.5 0.5 1.0]  GraphicAmbientColor=[0.15 0.15 0.15 1.0]  GraphicEmissiveColor=[0.0 0.0 0.0 1.0]  GraphicShininess=75  GraphicOpacity=cage_opc  GeometryShape=GeneralExtrusion  RectangleSize=[1 1]  RectangleSizeUnits=m  BrickDimensions=[1 1 1]  BrickDimensionUnits=m  CylinderRadius=1  CylinderRadiusUnits=m  CylinderLength=1  CylinderLengthUnits=m  SphereRadius=1  SphereRadiusUnits=m  EllipsoidRadii=[1 1 1]  EllipsoidRadiiUnits=m  ExtrusionCrossSection=cage_web_xc  ExtrusionCrossSectionUnits=m  ExtrusionLength=cage_web_thk  ExtrusionLengthUnits=m  PolygonNumSides=3  PolygonOuterRadius=1  PolygonOuterRadiusUnits=m  ExtGeomFileType=STEP  ExtGeomFileUnits=m  RevolutionCrossSection=[1 1; 1 -1; 2 -1; 2 1]  RevolutionCrossSectionUnits=m  RevolutionExtent=Full  RevolutionAngle=180  RevolutionAngleUnits=deg
  B : PMIOPort  Side=Left
  connections:
  B/RConn1 -- Transform Cage Loop/LConn1 -- Transform Web Ctrline/LConn1
  Loop/RConn1 -- Transform Cage Loop/RConn1
  Transform Web/LConn1 -- Transform Web Ctrline/RConn1
  Web/RConn1 -- Transform Web/RConn1

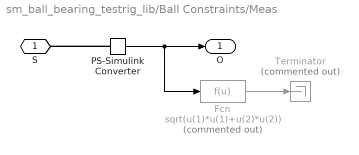
== system sm_ball_bearing_testrig_lib/Ball Constraints/Meas ==
  Fcn : Fcn  Commented=on  Expr=sqrt(u(1)*u(1)+u(2)*u(2))
  PS-Simulink Converter : nesl_utility/PS-Simulink Converter  PhysicalDomain=network_engine_domain  SubClassName=ps_output  LeftPortType=input  RightPortType=output  PseudoPeriodic=off  Frequencies=[]  Unit=1  AffineConversion=off
  Terminator : Terminator  Commented=on
  S : PMIOPort  Side=Left
  O : Outport
  wires:
  PS-Simulink Converter/1 -> Fcn/1, O/1
  Fcn/1 -> Terminator/1
  connections:
  PS-Simulink Converter/LConn1 -- S/RConn1

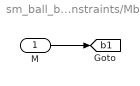
== system sm_ball_bearing_testrig_lib/Cage Constraints/Mb1 ==
  M : Inport
  tag scope: b1=global
  wires:
  M/1 -> [b1]

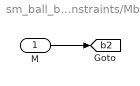
== system sm_ball_bearing_testrig_lib/Cage Constraints/Mb2 ==
  M : Inport
  tag scope: b2=global
  wires:
  M/1 -> [b2]

== system sm_ball_bearing_testrig_lib/Cage Constraints/Mb3 ==
  M : Inport
  tag scope: b3=global
  wires:
  M/1 -> [b3]

== system sm_ball_bearing_testrig_lib/Cage Constraints/Mb4 ==
  M : Inport
  tag scope: b4=global
  wires:
  M/1 -> [b4]

== system sm_ball_bearing_testrig_lib/Cage Constraints/Mb5 ==
  M : Inport
  tag scope: b5=global
  wires:
  M/1 -> [b5]

== system sm_ball_bearing_testrig_lib/Cage Constraints/Mb6 ==
  M : Inport
  tag scope: b6=global
  wires:
  M/1 -> [b6]

== system sm_ball_bearing_testrig_lib/Cage Constraints/Mb7 ==
  M : Inport
  tag scope: b7=global
  wires:
  M/1 -> [b7]

== system sm_ball_bearing_testrig_lib/Cage Constraints/Mb8 ==
  M : Inport
  tag scope: b8=global
  wires:
  M/1 -> [b8]

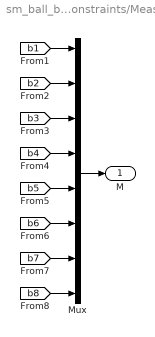
== system sm_ball_bearing_testrig_lib/Cage Constraints/Meas ==
  Mux : Mux  Inputs=8
  M : Outport
  wires:
  [b8] -> Mux/8
  [b7] -> Mux/7
  [b6] -> Mux/6
  [b5] -> Mux/5
  [b4] -> Mux/4
  [b3] -> Mux/3
  [b2] -> Mux/2
  [b1] -> Mux/1
  Mux/1 -> M/1

== system sm_ball_bearing_testrig_lib/Cage Forces/Mb1 ==
  M : Inport
  tag scope: b1=global
  wires:
  M/1 -> [b1]

== system sm_ball_bearing_testrig_lib/Cage Forces/Mb2 ==
  M : Inport
  tag scope: b2=global
  wires:
  M/1 -> [b2]

== system sm_ball_bearing_testrig_lib/Cage Forces/Mb3 ==
  M : Inport
  tag scope: b3=global
  wires:
  M/1 -> [b3]

== system sm_ball_bearing_testrig_lib/Cage Forces/Mb4 ==
  M : Inport
  tag scope: b4=global
  wires:
  M/1 -> [b4]

== system sm_ball_bearing_testrig_lib/Cage Forces/Mb5 ==
  M : Inport
  tag scope: b5=global
  wires:
  M/1 -> [b5]

== system sm_ball_bearing_testrig_lib/Cage Forces/Mb6 ==
  M : Inport
  tag scope: b6=global
  wires:
  M/1 -> [b6]

== system sm_ball_bearing_testrig_lib/Cage Forces/Mb7 ==
  M : Inport
  tag scope: b7=global
  wires:
  M/1 -> [b7]

== system sm_ball_bearing_testrig_lib/Cage Forces/Mb8 ==
  M : Inport
  tag scope: b8=global
  wires:
  M/1 -> [b8]

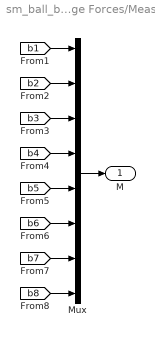
== system sm_ball_bearing_testrig_lib/Cage Forces/Meas ==
  Mux : Mux  Inputs=8
  M : Outport
  wires:
  [b8] -> Mux/8
  [b7] -> Mux/7
  [b6] -> Mux/6
  [b5] -> Mux/5
  [b4] -> Mux/4
  [b3] -> Mux/3
  [b2] -> Mux/2
  [b1] -> Mux/1
  Mux/1 -> M/1
